simulink library "helperCoordinateTransformLib"  (R2020a)
settings: Solver=VariableStepAuto  StartTime=0.0  StopTime=10.0  RelTol=1e-3
values from neighbouring files (symbols this model uses):
  scenario = drivingScenario    [helperGetLaneFollowingScenario.m]
settings Model: Creator=The MathWorks, Inc.  LastModifiedBy=The MathWorks, Inc.
settings DebuggingCC: SymbolicDimsDataTypeCodeGenerationDiagnostic=none

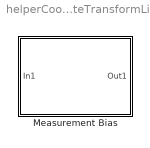
== system helperCoordinateTransformLib ==
  Measurement Bias : Subsystem  mask(Measurement Bias){offsetPositionX=scenario.Actors(1).Length/2 - scenario.Actors(1).RearOverhang}
      mask prompts: offsetPositionX "Offset to add to position x"
      mask help: Biases the position measurement. The first element of the measurement must be position.
      settings: AttributesFormatString=|
      | --------------------------------------
      | offsetPositionX = %<offsetPositionX>
      mask Display: disp(["Measurement","Bias"])

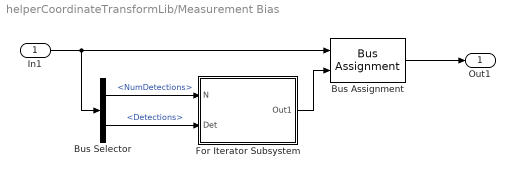
== system helperCoordinateTransformLib/Measurement Bias ==
  In1 : Inport
  Bus Assignment : BusAssignment  AssignedSignals=Detections
  Bus Selector : BusSelector  OutputSignals=NumDetections,Detections
  For Iterator Subsystem : Subsystem  TreatAsAtomicUnit=on
  Out1 : Outport  VectorParamsAs1DForOutWhenUnconnected=off
  wires:
  Bus Selector/1 -> For Iterator Subsystem/1(N)  "<NumDetections>"
  In1/1 -> Bus Assignment/1, Bus Selector/1
  Bus Selector/2 -> For Iterator Subsystem/2(Det)  "<Detections>"
  Bus Assignment/1 -> Out1/1
  For Iterator Subsystem/1(Out1) -> Bus Assignment/2

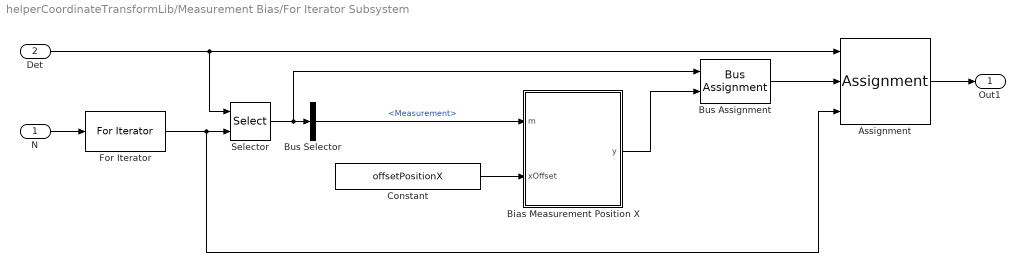
== system helperCoordinateTransformLib/Measurement Bias/For Iterator Subsystem ==
  N : Inport
  Det : Inport  Port=2
  Assignment : Assignment  DiagnosticForDimensions=Warning  IndexOptions=Index vector (port)  Indices=1  OutputSizes=1
  Bias Measurement Position X : MATLAB Function  TreatAsAtomicUnit=on
  Bus Assignment : BusAssignment  AssignedSignals=Measurement
  Bus Selector : BusSelector  OutputSignals=Measurement
  Constant : Constant  Value=offsetPositionX
  For Iterator : ForIterator  IterationSource=external
  Selector : Selector  IndexOptions=Index vector (port)  Indices=[1 3]  OutputSizes=1
  Out1 : Outport  VectorParamsAs1DForOutWhenUnconnected=off
  wires:
  N/1 -> For Iterator/1
  For Iterator/1 -> Assignment/3, Selector/2
  Assignment/1 -> Out1/1
  Det/1 -> Selector/1, Assignment/1
  Selector/1 -> Bus Assignment/1, Bus Selector/1
  Bus Assignment/1 -> Assignment/2
  Bus Selector/1 -> Bias Measurement Position X/1(m)  "<Measurement>"
  Bias Measurement Position X/1(y) -> Bus Assignment/2
  Constant/1 -> Bias Measurement Position X/2(xOffset)

== matlab function helperCoordinateTransformLib/Measurement Bias/For Iterator Subsystem/Bias Measurement Position X ==
  data: m input; y output; xOffset input
function y = fcn(m, xOffset)

y = m;
y(1) = y(1) + xOffset;
